simulink model "lab5_model"  (R2015a)
settings: Solver=ode45  StartTime=0.0  StopTime=20  RelTol=1e-3
values from neighbouring files (symbols this model uses):
  A = [0 1 0 0;(-K/M1) (-D_M/M1) (K/M1) 0;0 0 0 1;(K/M2) 0 (-K/M2) 0]    [lab5.m]
  B = [0;0;0;(1/M2)]    [lab5.m]
  C = [0 0 0 1]    [lab5.m]
  D = [0]    [lab5.m]
  D_M = 52    [lab5.m]
  K = 100    [lab5.m]
  M1 = 1    [lab5.m]
  M2 = 1.5    [lab5.m]
settings Model: Creator=Jessica  LastModifiedBy=Jessica

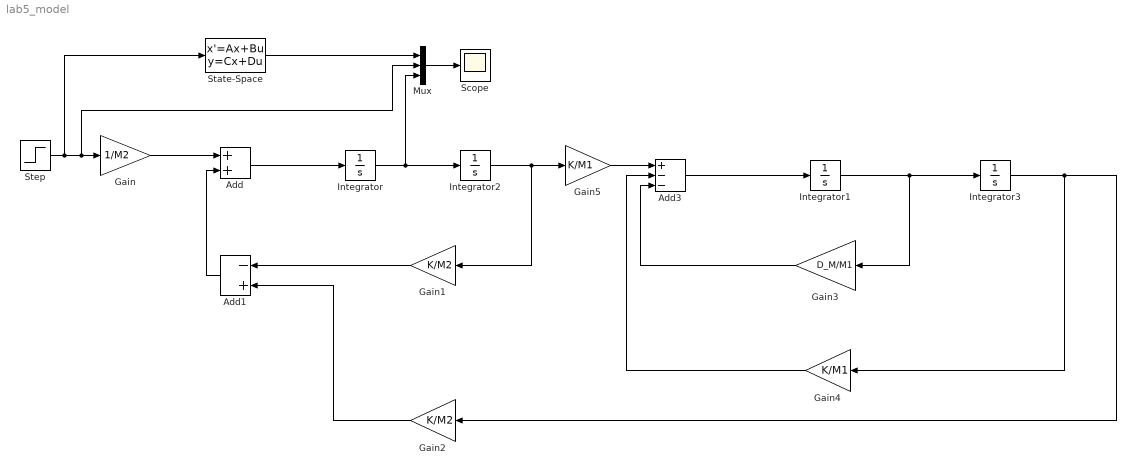
== system lab5_model ==
  Add : Sum
  Add1 : Sum  Inputs=-+
  Add3 : Sum  Inputs=+--
  Gain : Gain  Gain=1/M2
  Gain1 : Gain  Gain=K/M2
  Gain2 : Gain  Gain=K/M2
  Gain3 : Gain  Gain=D_M/M1
  Gain4 : Gain  Gain=K/M1
  Gain5 : Gain  Gain=K/M1
  Integrator{,1..3} (4 alike) : Integrator
  Mux : Mux  Inputs=3
  Scope : Scope
      settings: SaveName=y
  State-Space : StateSpace  A=A  B=B  C=C  D=D  X0=0
  Step : Step  Before=1  After=0  SampleTime=0
  wires:
  Gain/1 -> Add/1
  Add1/1 -> Add/2
  Add/1 -> Integrator/1
  Gain1/1 -> Add1/1
  Gain2/1 -> Add1/2
  Add3/1 -> Integrator1/1
  Integrator1/1 -> Gain3/1, Integrator3/1
  Integrator3/1 -> Gain2/1, Gain4/1
  Gain5/1 -> Add3/1
  Integrator2/1 -> Gain1/1, Gain5/1
  Integrator/1 -> Mux/3, Integrator2/1
  Step/1 -> Mux/2, Gain/1, State-Space/1
  Mux/1 -> Scope/1
  State-Space/1 -> Mux/1
  Gain3/1 -> Add3/3
  Gain4/1 -> Add3/2
